simulink model "CoolingCheese_3rdPoint"  (R2022a)
settings: Solver=VariableStepAuto  StartTime=0.0  StopTime=H  RelTol=1e-3
undefined symbols (not defined in the file): C_c, C_f, k_af, k_fc, q_star, Ts, var_wc, var_wf
settings Model: Creator=mrnel  LastModifiedBy=mrnel

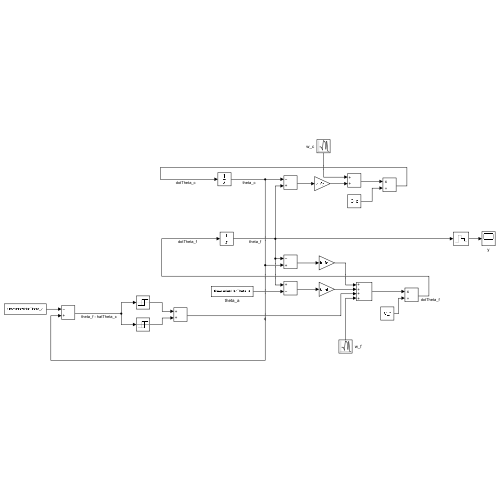
[thumbnail: Simulink's stored preview of the top-level diagram]
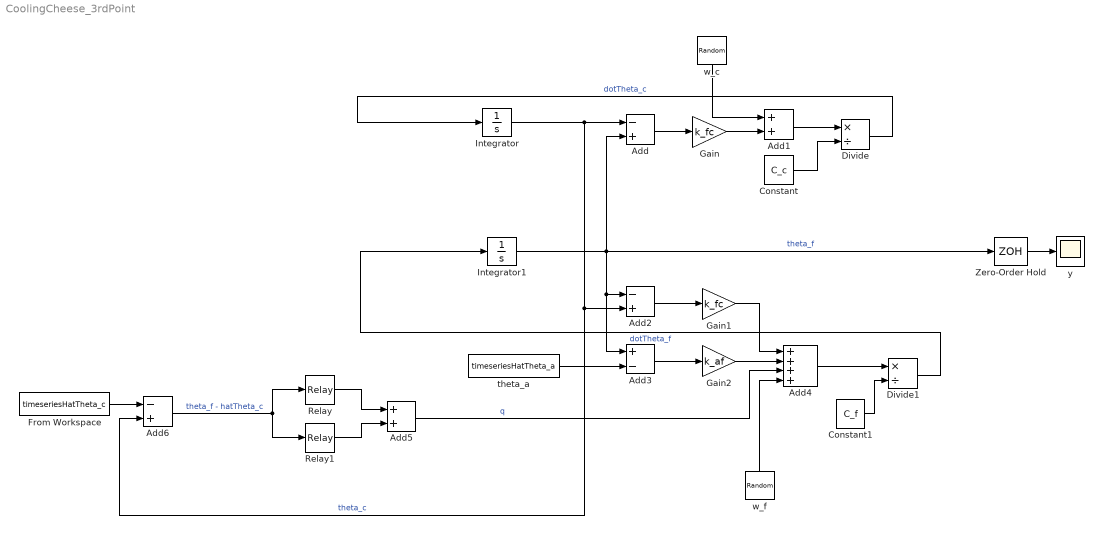
== system CoolingCheese_3rdPoint ==
  Add : Sum  Inputs=-+
  Add1 : Sum
  Add2 : Sum  Inputs=-+
  Add3 : Sum  Inputs=+-
  Add4 : Sum  Inputs=++++
  Add5 : Sum
  Add6 : Sum  Inputs=-+
  Constant : Constant  Value=C_c
  Constant1 : Constant  Value=C_f
  Divide : Product  Inputs=*/
  Divide1 : Product  Inputs=*/
  From Workspace : FromWorkspace  VariableName=timeseriesHatTheta_c  SampleTime=Ts
  Gain : Gain  Gain=k_fc
  Gain1 : Gain  Gain=k_fc
  Gain2 : Gain  Gain=k_af
  Integrator : Integrator
  Integrator1 : Integrator
  Relay : Relay  OnSwitchValue=2  OffSwitchValue=2  OnOutputValue=-q_star/2  OffOutputValue=q_star/2
  Relay1 : Relay  OnSwitchValue=-2  OffSwitchValue=-2  OnOutputValue=-q_star/2  OffOutputValue=q_star/2
  Zero-Order Hold : ZeroOrderHold  SampleTime=Ts
  theta_a : FromWorkspace  VariableName=timeseriesHatTheta_a  SampleTime=Ts
  w_c : RandomNumber  Variance=var_wc  SampleTime=Ts
  w_f : RandomNumber  Variance=var_wf  SampleTime=Ts
  y : Scope
  wires:
  Divide/1 -> Integrator/1  "dotTheta_c"
  Integrator/1 -> Add6/2, Add2/2, Add/1  "theta_c"
  Integrator1/1 -> Zero-Order Hold/1, Add3/1, Add2/1, Add/2  "theta_f"
  Add/1 -> Gain/1
  Gain/1 -> Add1/2
  w_c/1 -> Add1/1
  Add1/1 -> Divide/1
  Constant/1 -> Divide/2
  Add2/1 -> Gain1/1
  theta_a/1 -> Add3/2
  Add3/1 -> Gain2/1
  Add5/1 -> Add4/3  "q"
  Gain2/1 -> Add4/2
  Gain1/1 -> Add4/1
  Add4/1 -> Divide1/1
  Constant1/1 -> Divide1/2
  Divide1/1 -> Integrator1/1  "dotTheta_f"
  w_f/1 -> Add4/4
  Zero-Order Hold/1 -> y/1
  Relay/1 -> Add5/1
  Relay1/1 -> Add5/2
  From Workspace/1 -> Add6/1
  Add6/1 -> Relay1/1, Relay/1  "theta_f - hatTheta_c"
